simulink model "sampleModel1800"  (R2023a)
settings: Solver=VariableStepAuto  StartTime=0.0  StopTime=10.0  RelTol=1e-3
libraries: hdlsllib x1, simulink x1
settings Model: Creator=user1  LastModifiedBy=user1

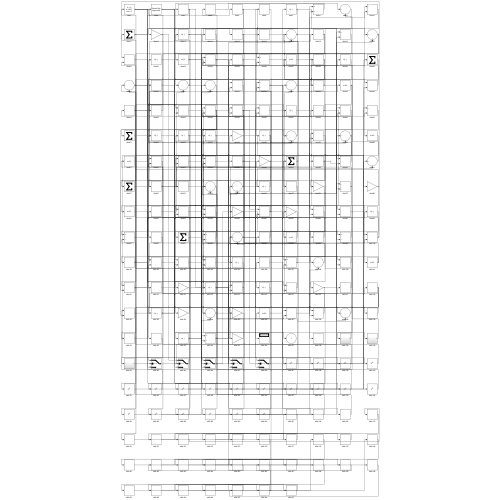
[thumbnail: Simulink's stored preview of the top-level diagram]
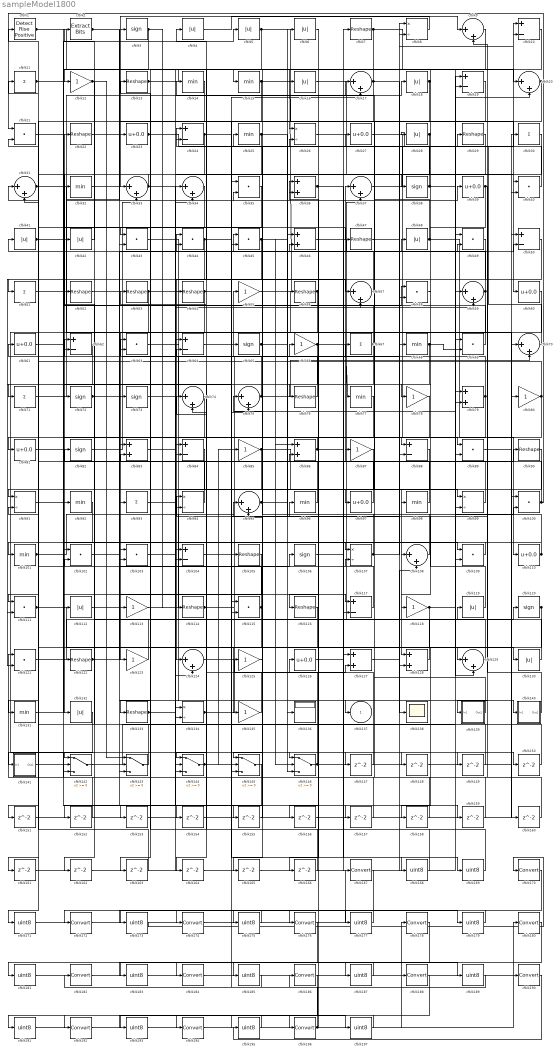
== system sampleModel1800 ==
  cfblk1 : hdlsllib/Logic and Bit Operations/Detect Rise Positive  vinit=0  OutDataTypeStr=boolean
  cfblk{10,19,24,50,62,64,84,88,104,117} (10 alike) : Sum  Inputs=+-
  cfblk{21,35,40,43..45,49,58,63,69,89,100,102..103,109,111,115,121} (18 alike) : DotProduct  OutDataTypeStr=Inherit: Inherit via internal rule
  cfblk{14..15,25,32,68,77,92,96,98,101,131} (11 alike) : MinMax
  cfblk{7,13,22,29,47,52..54,56,76,90,105,114,116,122,133} (16 alike) : Reshape
  cfblk{3,38,65,72..73,82,106,120} (8 alike) : Signum
  cfblk{8,26,91,94,99,107,134} (7 alike) : Product  Inputs=*/  RndMeth=Zero  SaturateOnIntegerOverflow=on
  cfblk{9,17,20,31,33..34,37,57,59,70,74..75,95,108,124,129} (16 alike) : Sum  Inputs=|++
  cfblk{11,30,51,67,71,93} (6 alike) : Sum  Inputs=+
  cfblk{23,27,39,60..61,81,97,110,126} (9 alike) : Bias  Bias=0.0  SaturateOnIntegerOverflow=off
  cfblk{4..6,16,18,28,41..42,48,112,119,130,132} (13 alike) : Abs  SaturateOnIntegerOverflow=off
  cfblk{12,55,66,78,80,85,87,113,118,123,125,135} (12 alike) : Gain
  cfblk{36,46,79,83,86,127..128} (7 alike) : Sum
  cfblk136 : Display
  cfblk138 : Scope
  cfblk139 : Subsystem
      settings: LibrarySourceBlock=|
      | hdlsllib/Ports &
      | Subsystems/Subsystem
  cfblk140 : Subsystem
      settings: LibrarySourceBlock=|
      | hdlsllib/Ports &
      | Subsystems/Subsystem
  cfblk141 : Subsystem
      settings: LibrarySourceBlock=|
      | hdlsllib/Ports &
      | Subsystems/Subsystem
  cfblk{142..146} (5 alike) : Switch  SaturateOnIntegerOverflow=off  InputSameDT=off
  cfblk{147..166} (20 alike) : Delay  SampleTime=1
  cfblk{167,170,172,174,176,178,180,182,184,186,188,190,192,194,196} (15 alike) : DataTypeConversion  SaturateOnIntegerOverflow=off  RndMeth=Floor
  cfblk{168..169,171,173,175,177,179,181,183,185,187,189,191,193,195,197} (16 alike) : DataTypeConversion  OutDataTypeStr=uint8  SaturateOnIntegerOverflow=off  RndMeth=Floor
  cfblk2 : simulink/Logic and Bit Operations/Extract Bits  bitsToExtract=Upper half  numBits=8  bitIdxRange=[0 7]  outScalingMode=Preserve fixed-point scaling
      settings: LibrarySourceBlock=|
      | hdlsllib/Logic and Bit
      | Operations/Extract Bits
  cfblk137 : Outport  VectorParamsAs1DForOutWhenUnconnected=off
  wires:
  cfblk98/1 -> cfblk37/1
  cfblk27/1 -> cfblk89/1
  cfblk111/1 -> cfblk129/1, cfblk86/2
  cfblk5/1 -> cfblk60/1, cfblk54/1, cfblk23/1
  cfblk67/1 -> cfblk36/2, cfblk164/1
  cfblk53/1 -> cfblk142/1, cfblk105/1
  cfblk84/1 -> cfblk123/1
  cfblk39/1 -> cfblk121/1, cfblk98/1
  cfblk8/1 -> cfblk33/1
  cfblk70/1 -> cfblk28/1
  cfblk76/1 -> cfblk61/1
  cfblk48/1 -> cfblk110/1, cfblk14/1
  cfblk63/1 -> cfblk140/1(In1)
  cfblk71/1 -> cfblk18/1
  cfblk29/1 -> cfblk132/1
  cfblk134/1 -> cfblk66/1, cfblk57/2
  cfblk60/1 -> cfblk112/1
  cfblk25/1 -> cfblk43/2, cfblk150/1
  cfblk14/1 -> cfblk113/1
  cfblk132/1 -> cfblk141/1(In1)
  cfblk45/1 -> cfblk86/1, cfblk84/2, cfblk145/3, cfblk148/1
  cfblk2/1 -> cfblk117/2, cfblk26/1, cfblk154/1
  cfblk44/1 -> cfblk124/1, cfblk121/2, cfblk17/2, cfblk143/3
  cfblk69/1 -> cfblk22/1
  cfblk55/1 -> cfblk100/1
  cfblk112/1 -> cfblk48/1
  cfblk62/1 -> cfblk92/1
  cfblk43/1 -> cfblk88/1
  cfblk51/1 -> cfblk39/1
  cfblk82/1 -> cfblk33/2
  cfblk108/1 -> cfblk75/1
  cfblk121/1 -> cfblk37/2
  cfblk7/1 -> cfblk69/1, cfblk125/1
  cfblk91/1 -> cfblk58/1
  cfblk3/1 -> cfblk12/1, cfblk114/1, cfblk143/2
  cfblk88/1 -> cfblk128/1
  cfblk140/1(Out1) -> cfblk94/1
  cfblk113/1 -> cfblk19/1
  cfblk38/1 -> cfblk24/1, cfblk20/2
  cfblk56/1 -> cfblk103/1, cfblk144/3
  cfblk66/1 -> cfblk77/1, cfblk111/2
  cfblk15/1 -> cfblk56/1, cfblk144/2, cfblk122/1
  cfblk135/1 -> cfblk82/1
  cfblk32/1 -> cfblk64/1
  cfblk120/1 -> cfblk144/1, cfblk158/1, cfblk161/1
  cfblk78/1 -> cfblk93/1
  cfblk86/1 -> cfblk83/1, cfblk36/1, cfblk109/1
  cfblk110/1 -> cfblk63/1, cfblk104/1
  cfblk1/1 -> cfblk79/2, cfblk47/1, cfblk75/2, cfblk115/2
  cfblk79/1 -> cfblk133/1, cfblk65/1
  cfblk35/1 -> cfblk72/1
  cfblk37/1 -> cfblk10/1
  cfblk58/1 -> cfblk118/1
  cfblk94/1 -> cfblk62/1
  cfblk23/1 -> cfblk29/1, cfblk38/1
  cfblk73/1 -> cfblk8/1
  cfblk16/1 -> cfblk129/2
  cfblk95/1 -> cfblk46/1, cfblk130/1
  cfblk127/1 -> cfblk119/1
  cfblk101/1 -> cfblk59/1, cfblk117/1
  cfblk59/1 -> cfblk88/2, cfblk17/1, cfblk73/1
  cfblk31/1 -> cfblk80/1, cfblk84/1
  cfblk61/1 -> cfblk5/1
  cfblk26/1 -> cfblk68/1
  cfblk11/1 -> cfblk20/1, cfblk155/1
  cfblk109/1 -> cfblk102/1
  cfblk75/1 -> cfblk70/2, cfblk64/2
  cfblk133/1 -> cfblk50/2, cfblk59/2
  cfblk52/1 -> cfblk63/2
  cfblk9/1 -> cfblk108/1
  cfblk18/1 -> cfblk97/1, cfblk45/2
  cfblk65/1 -> cfblk136/1, cfblk146/2
  cfblk30/1 -> cfblk116/1
  cfblk126/1 -> cfblk120/1
  cfblk119/1 -> cfblk95/1
  cfblk17/1 -> cfblk40/1, cfblk94/2, cfblk16/1
  cfblk50/1 -> cfblk81/1
  cfblk4/1 -> cfblk9/1
  cfblk46/1 -> cfblk49/2
  cfblk124/1 -> cfblk127/2
  cfblk40/1 -> cfblk4/1
  cfblk143/1 -> cfblk62/2
  cfblk122/1 -> cfblk106/1, cfblk90/1
  cfblk128/1 -> cfblk83/2
  cfblk28/1 -> cfblk128/2, cfblk51/1
  cfblk93/1 -> cfblk35/2
  cfblk64/1 -> cfblk55/1
  cfblk49/1 -> cfblk78/1
  cfblk97/1 -> cfblk31/1
  cfblk54/1 -> cfblk71/1, cfblk26/2
  cfblk100/1 -> cfblk21/1, cfblk45/1
  cfblk33/1 -> cfblk32/1, cfblk99/2
  cfblk114/1 -> cfblk6/1, cfblk146/3, cfblk168/1
  cfblk107/1 -> cfblk44/1, cfblk10/2
  cfblk20/1 -> cfblk145/1, cfblk104/2
  cfblk21/1 -> cfblk43/1
  cfblk42/1 -> cfblk2/1
  cfblk24/1 -> cfblk103/2, cfblk109/2, cfblk89/2
  cfblk130/1 -> cfblk9/2
  cfblk57/1 -> cfblk41/1
  cfblk142/1 -> cfblk19/2
  cfblk123/1 -> cfblk52/1
  cfblk6/1 -> cfblk76/1
  cfblk72/1 -> cfblk34/1, cfblk67/1
  cfblk10/1 -> cfblk134/2
  cfblk115/1 -> cfblk31/2, cfblk162/1
  cfblk81/1 -> cfblk107/1
  cfblk131/1 -> cfblk87/1
  cfblk141/1(Out1) -> cfblk145/2
  cfblk116/1 -> cfblk135/1
  cfblk34/1 -> cfblk101/1
  cfblk96/1 -> cfblk24/2
  cfblk102/1 -> cfblk137/1
  cfblk80/1 -> cfblk139/1(In1), cfblk21/2
  cfblk77/1 -> cfblk142/3
  cfblk85/1 -> cfblk111/1, cfblk138/1
  cfblk13/1 -> cfblk15/1, cfblk57/1
  cfblk68/1 -> cfblk69/2, cfblk156/1
  cfblk139/1(Out1) -> cfblk27/1
  cfblk104/1 -> cfblk58/2
  cfblk47/1 -> cfblk8/2
  cfblk129/1 -> cfblk102/2
  cfblk19/1 -> cfblk91/1
  cfblk144/1 -> cfblk96/1, cfblk85/1
  cfblk36/1 -> cfblk99/1, cfblk149/1
  cfblk117/1 -> cfblk11/1
  cfblk118/1 -> cfblk100/2, cfblk131/1
  cfblk41/1 -> cfblk3/1, cfblk146/1
  cfblk146/1 -> cfblk53/1, cfblk30/1
  cfblk99/1 -> cfblk25/1
  cfblk12/1 -> cfblk42/1, cfblk143/1
  cfblk83/1 -> cfblk147/1
  cfblk147/1 -> cfblk46/2
  cfblk148/1 -> cfblk70/1
  cfblk149/1 -> cfblk91/2
  cfblk150/1 -> cfblk35/1
  cfblk92/1 -> cfblk151/1
  cfblk151/1 -> cfblk79/1
  cfblk145/1 -> cfblk152/1
  cfblk152/1 -> cfblk142/2
  cfblk87/1 -> cfblk153/1
  cfblk153/1 -> cfblk124/2
  cfblk154/1 -> cfblk50/1
  cfblk155/1 -> cfblk95/2
  cfblk156/1 -> cfblk40/2
  cfblk22/1 -> cfblk157/1
  cfblk157/1 -> cfblk44/2
  cfblk158/1 -> cfblk134/1
  cfblk103/1 -> cfblk159/1
  cfblk159/1 -> cfblk127/1
  cfblk89/1 -> cfblk160/1
  cfblk160/1 -> cfblk107/2
  cfblk161/1 -> cfblk108/2
  cfblk162/1 -> cfblk34/2
  cfblk105/1 -> cfblk163/1
  cfblk163/1 -> cfblk1/1
  cfblk164/1 -> cfblk49/1
  cfblk125/1 -> cfblk165/1
  cfblk165/1 -> cfblk7/1
  cfblk90/1 -> cfblk166/1
  cfblk166/1 -> cfblk13/1
  cfblk168/1 -> cfblk74/1
  cfblk106/1 -> cfblk169/1
  cfblk169/1 -> cfblk74/2
  cfblk74/1 -> cfblk171/1
  cfblk171/1 -> cfblk167/1
  cfblk167/1 -> cfblk173/1
  cfblk173/1 -> cfblk170/1
  cfblk170/1 -> cfblk175/1
  cfblk175/1 -> cfblk172/1
  cfblk172/1 -> cfblk177/1
  cfblk177/1 -> cfblk174/1
  cfblk174/1 -> cfblk179/1
  cfblk179/1 -> cfblk176/1
  cfblk176/1 -> cfblk181/1
  cfblk181/1 -> cfblk178/1
  cfblk178/1 -> cfblk183/1
  cfblk183/1 -> cfblk180/1
  cfblk180/1 -> cfblk185/1
  cfblk185/1 -> cfblk182/1
  cfblk182/1 -> cfblk187/1
  cfblk187/1 -> cfblk184/1
  cfblk184/1 -> cfblk189/1
  cfblk189/1 -> cfblk186/1
  cfblk186/1 -> cfblk191/1
  cfblk191/1 -> cfblk188/1
  cfblk188/1 -> cfblk193/1
  cfblk193/1 -> cfblk190/1
  cfblk194/1 -> cfblk196/1
  cfblk190/1 -> cfblk195/1
  cfblk195/1 -> cfblk192/1
  cfblk196/1 -> cfblk115/1, cfblk126/1
  cfblk192/1 -> cfblk197/1
  cfblk197/1 -> cfblk194/1

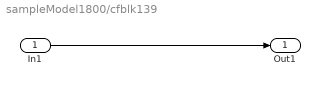
== system sampleModel1800/cfblk139 ==
  In1 : Inport
  Out1 : Outport
  wires:
  In1/1 -> Out1/1

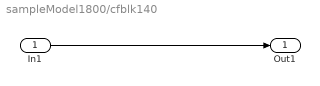
== system sampleModel1800/cfblk140 ==
  In1 : Inport
  Out1 : Outport
  wires:
  In1/1 -> Out1/1

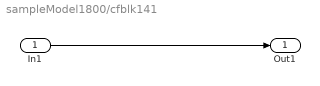
== system sampleModel1800/cfblk141 ==
  In1 : Inport
  Out1 : Outport
  wires:
  In1/1 -> Out1/1
